simulink model "PSO_MPPT"  (Simulink 10.2)
settings: Solver=FixedStepAuto  StartTime=0.0  StopTime=0.3  FixedStep=1e-6  RelTol=1e-3
undefined symbols (not defined in the file): L
libraries: powerlib x16, re_lib x4, powerlib_meascontrol x1
settings Model: Creator=11383  LastModifiedBy=YiboWang  SimulationMode=accelerator
settings DataIOCC: SaveFormat=Dataset  SignalLoggingSaveFormat=Dataset
settings OptimizationCC: LifeSpan=auto
settings DebuggingCC: UnderspecifiedInitializationDetection=Simplified  MergeDetectMultiDrivingBlocksExec=error  FcnCallInpInsideContextMsg=error  SFUnexpectedBacktrackingDiag=error  SFNoUnconditionalDefaultTransitionDiag=error  SFExecutionAtInitializationDiag=warning
settings HardwareCC: ProdBitPerPointer=64  ProdBitPerSizeT=64  ProdBitPerPtrDiffT=64  ProdLargestAtomicFloat=Float  ProdIntDivRoundTo=Zero  ProdEndianess=LittleEndian  ProdWordSize=64  ProdHWDeviceType=Intel->x86-64 (Windows64)
settings ModelReferenceCC: PropagateSignalLabelsOutOfModel=on
settings GRTTargetCC: TargetLangStandard=C99 (ISO)  CombineOutputUpdateFcns=on  GRTInterface=off
settings ConfigComp: CovMetricSettings=dwe  CovSaveCumulativeToWorkspaceVar=off  CovSaveSingleToWorkspaceVar=off  CovExternalEMLEnable=on
settings SimscapeCC: SimscapeNormalizeSystem=off

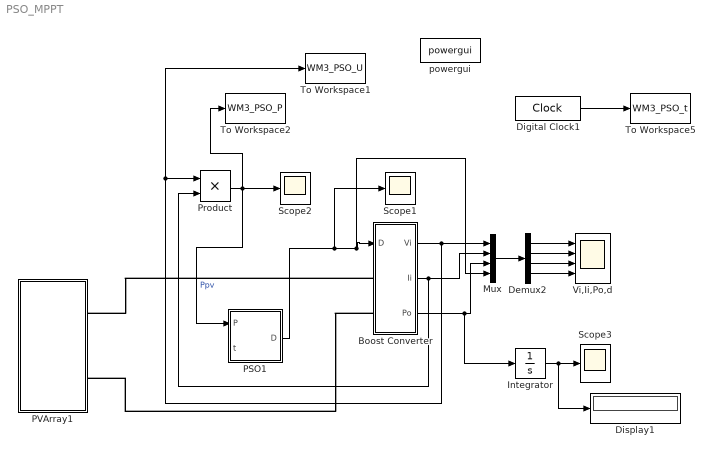
== system PSO_MPPT ==
  Boost Converter : Subsystem
  Demux2 : Demux
  Digital Clock1 : DigitalClock  SampleTime=-1
  Display1 : Display
  Integrator : Integrator
  Mux : Mux
  PSO1 : MATLAB Function  TreatAsAtomicUnit=on  SystemSampleTime=0.005
  PVArray1 : Subsystem
  Product : Product
  Scope1 : Scope
  Scope2 : Scope
  Scope3 : Scope
  To Workspace1 : ToWorkspace  VariableName=WM3_PSO_U  SampleTime=-1
  To Workspace2 : ToWorkspace  VariableName=WM3_PSO_P  SampleTime=-1
  To Workspace5 : ToWorkspace  VariableName=WM3_PSO_t  SampleTime=-1
  Vi,Ii,Po,d : Scope  NumInputPorts=4
  powergui : powerlib/powergui  SimulationMode=Discrete  SampleTime=1e-6  frequency=60  Iterations=50  frequencyindice=0  Pbase=100e6  ErrMax=1e-4  UnitsV=kV  UnitsW=MW  buscounter=0  FunctionMessages=off  echomessages=off  EnableUseOfTLC=off  CurrentSourceSwitches=off  DisableSnubberDevices=off  DisableRonSwitches=off  DisableVfSwitches=off  DisplayEquations=off  AutomaticDiscreteSolvers=off  SolverType=Tustin  Interpol=off  ExternalGateDelay=off  methode=off  Ts=0  x0status=blocks  SPID=off  SwTol=0  HookPort=off  NonlinearTolerance=0  nMaxIteration=15  ContinueOnMaxIteration=off  RestoreLinks=warning  ResistiveCurrentMeasurement=off  Frange=[0:2:500]  Ylog=off  Xlog=on  ShowGrid=off  save=off  variable=ZData  structure=0  ZoomFFT=on  StartTime=0.0  cycles=1  DisplayStyle=1  fundamental=60  FreqAxis=off  MaxFrequency=1000  frequencyindicesteady=1  RmsSteady=1  display=off
  wires:
  Digital Clock1/1 -> To Workspace5/1
  Demux2/1 -> Vi,Ii,Po,d/1
  Demux2/2 -> Vi,Ii,Po,d/2
  Demux2/3 -> Vi,Ii,Po,d/3
  Demux2/4 -> Vi,Ii,Po,d/4
  Boost Converter/1(Vi) -> Mux/1, To Workspace1/1, Product/1
  Boost Converter/2(Ii) -> Mux/2, Product/2
  Boost Converter/3(Po) -> Integrator/1, Mux/3
  PSO1/1(D) -> Scope1/1, Mux/4, Boost Converter/1(D)
  Product/1 -> PSO1/1(P), To Workspace2/1, Scope2/1  "Ppv"
  Mux/1 -> Demux2/1
  Integrator/1 -> Display1/1, Scope3/1
  connections:
  Boost Converter/LConn2 -- PVArray1/RConn2
  Boost Converter/LConn1 -- PVArray1/RConn1

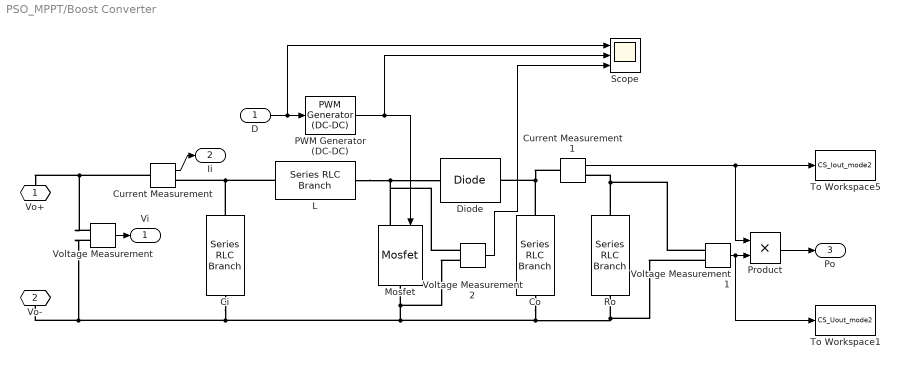
== system PSO_MPPT/Boost Converter ==
  D : Inport
  Ci : powerlib/Elements/Series RLC Branch  LConnTagsString=__new0  RConnTagsString=__new0  BranchType=C  Resistance=1  Inductance=L  SetiL0=off  InitialCurrent=0  Capacitance=10e-5  Setx0=off  InitialVoltage=0  Measurements=None
  Co : powerlib/Elements/Series RLC Branch  LConnTagsString=__new0  RConnTagsString=__new0  BranchType=C  Resistance=1  Inductance=L  SetiL0=off  InitialCurrent=0  Capacitance=9e-05  Setx0=off  InitialVoltage=0  Measurements=None
  Current Measurement : powerlib/Measurements/Current Measurement  PhasorSimulation=off  OutputType=Complex  PSBequivalent=0
  Current Measurement1 : powerlib/Measurements/Current Measurement  PhasorSimulation=off  OutputType=Complex  PSBequivalent=0
  Diode : powerlib/Power Electronics/Diode  Ron=0.001  Lon=0  Vf=0.8  IC=0  UseSnubber=off  Rs=inf  Cs=250e-9  Measurements=off
  L : powerlib/Elements/Series RLC Branch  LConnTagsString=__new0  RConnTagsString=__new0  BranchType=L  Resistance=1  Inductance=2e-3  SetiL0=off  InitialCurrent=0  Capacitance=1e-6  Setx0=off  InitialVoltage=0  Measurements=None
  Mosfet : powerlib/Power Electronics/Mosfet  Ron=0.1  Lon=0  Rd=0.01  Vfd=0  IC=0  Rs=1e5  Cs=inf  Measurements=off
  PWM Generator (DC-DC) : powerlib_meascontrol/Pulse & Signal Generators/PWM Generator (DC-DC)  Fsw=10000  Ts=0
  Product : Product
  Ro : powerlib/Elements/Series RLC Branch  LConnTagsString=__new0  RConnTagsString=__new0  BranchType=R  Resistance=33  Inductance=L  SetiL0=off  InitialCurrent=0  Capacitance=1e-6  Setx0=off  InitialVoltage=0  Measurements=None
  Scope : Scope  NumInputPorts=3
  To Workspace1 : ToWorkspace  VariableName=CS_Uout_mode2  SampleTime=-1
  To Workspace5 : ToWorkspace  VariableName=CS_Iout_mode2  SampleTime=-1
  Voltage Measurement : powerlib/Measurements/Voltage Measurement  PhasorSimulation=off  OutputType=Complex  PSBequivalent=0
  Voltage Measurement1 : powerlib/Measurements/Voltage Measurement  PhasorSimulation=off  OutputType=Complex  PSBequivalent=0
  Voltage Measurement2 : powerlib/Measurements/Voltage Measurement  PhasorSimulation=off  OutputType=Complex  PSBequivalent=0
  Vo+ : PMIOPort  Side=Left
  Vo- : PMIOPort  Port=2  Side=Left
  Vi : Outport  VectorParamsAs1DForOutWhenUnconnected=off
  Ii : Outport  Port=2  VectorParamsAs1DForOutWhenUnconnected=off
  Po : Outport  Port=3  VectorParamsAs1DForOutWhenUnconnected=off
  wires:
  Current Measurement1/1 -> To Workspace5/1, Product/1
  Product/1 -> Po/1
  Voltage Measurement1/1 -> To Workspace1/1, Product/2
  Current Measurement/1 -> Ii/1
  PWM Generator (DC-DC)/1 -> Scope/2, Mosfet/1
  D/1 -> Scope/1, PWM Generator (DC-DC)/1
  Voltage Measurement/1 -> Vi/1
  Voltage Measurement2/1 -> Scope/3
  connections:
  Current Measurement1/LConn1 -- Co/LConn1 -- Diode/RConn1
  L/RConn1 -- Voltage Measurement2/LConn1 -- Mosfet/LConn1 -- Diode/LConn1
  L/LConn1 -- Current Measurement/RConn1 -- Ci/LConn1
  Co/RConn1 -- Voltage Measurement1/LConn2 -- Ro/RConn1 -- Ci/RConn1 -- Vo-/RConn1 -- Voltage Measurement/LConn2 -- Voltage Measurement2/LConn2 -- Mosfet/RConn1
  Ro/LConn1 -- Voltage Measurement1/LConn1 -- Current Measurement1/RConn1
  Current Measurement/LConn1 -- Vo+/RConn1 -- Voltage Measurement/LConn1

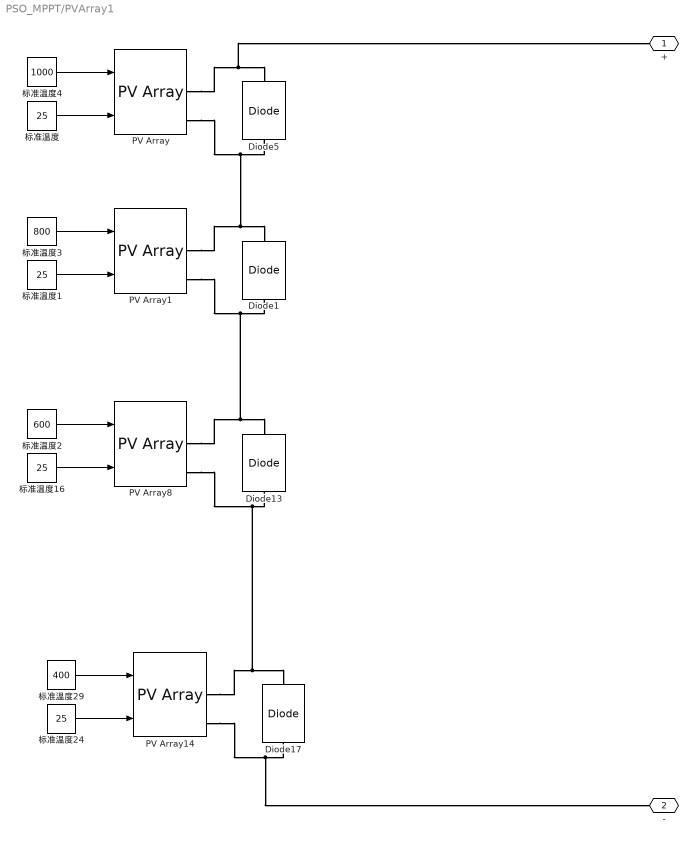
== system PSO_MPPT/PVArray1 ==
  Diode{1,5,13,17} (4 alike) : powerlib/Power Electronics/Diode  Ron=0.001  Lon=0  Vf=0.8  IC=0  UseSnubber=off  Rs=inf  Cs=250e-9  Measurements=off
  PV Array{,1,8,14} (4 alike) : re_lib/Solar/PV Array  Npar=1  Nser=1  PlotType=array @ 1000 W/m2 & specified temperatures  S_vec="[ 1000  500  100 ]"  Temp_C_vec="[ 45 25  ]"  ModuleName=User-defined  PlotWhenSelected=off  Pm=120.75  Ncell=16  Voc=22  Isc=7.5  Vm=17.5  Im=6.9  beta_Voc_pc=-0.36099  alpha_Isc_pc=0.102  beta_Voc=-0.079418  alpha_Isc=0.00765  IL=7.6829  I0=2.1898e-10  nI=2.2089  Rsh=50.0358  Rs=0.26399  RobustModel=off  RobustCellTemperature=313.3991  BAL=off  Tc=1e-6  Tfilter=5e-5
  标准温度{,1,16,24} (4 alike) : Constant  Value=25  SampleTime=0.001
  标准温度2 : Constant  Value=600  SampleTime=0.001
  标准温度29 : Constant  Value=400  SampleTime=0.001
  标准温度3 : Constant  Value=800  SampleTime=0.001
  标准温度4 : Constant  Value=1000  SampleTime=0.001
  + : PMIOPort  Side=Right
  - : PMIOPort  Port=2  Side=Right
  wires:
  标准温度16/1 -> PV Array8/2
  标准温度24/1 -> PV Array14/2
  标准温度29/1 -> PV Array14/1
  标准温度1/1 -> PV Array1/2
  标准温度/1 -> PV Array/2
  标准温度2/1 -> PV Array8/1
  标准温度3/1 -> PV Array1/1
  标准温度4/1 -> PV Array/1
  connections:
  Diode17/RConn1 -- PV Array14/RConn1 -- Diode13/LConn1 -- PV Array8/RConn2
  Diode5/RConn1 -- +/RConn1 -- PV Array/RConn1
  Diode5/LConn1 -- PV Array/RConn2 -- Diode1/RConn1 -- PV Array1/RConn1
  Diode17/LConn1 -- -/RConn1 -- PV Array14/RConn2
  Diode13/RConn1 -- PV Array8/RConn1 -- Diode1/LConn1 -- PV Array1/RConn2

== matlab function PSO1 ==
  data: D output double; P input double; t input double
function D=PSO(P,t)
%% 参数定义
w=0.5;                              %惯性权重
c1=0.5;                             %个体学习因子/加速度因子
c2=0.9;                             %群体学习因子/加速度因子
N=4;                                %粒子个数
pmin=0.1;                           %输出最小值
pmax=0.9;                             %输出最大值
r1=rand;
r2=rand;
%% Starting Up
persistent p;
if isempty(p) 
    %Create empty particle 定义空粒子属性
    %p.x=[0.1 0.25 0.4 0.55 0.7];
    %p.x=[0.1 0.3 0.5 0.7];
    p.x=[0.1,0.3,0.6,0.9];
    %p.x = linspace(0.4,0.6,N);
    %p.x = linspace(pmin,pmax,N);    %线性平均划分输出的最小最大差值成为N个数
    p.v = zeros(1,N);               %粒子速度初始化
    p.y = zeros(1,N);               %粒子位置对应值初始化
	p.bx = zeros(1,N);              %粒子最优位置初始化
    p.by = zeros(1,N);              %粒子最优值初始化
    p.bg=pmin;                      %全局最优值初始化
    p.k=1;                          %控制循环次数
    D=p.x(p.k);                     %输出值初始化
else
%% Input
p.y(p.k)=P;                         %存储输入的功率值到p.y中的第p.k个

%% Best Particle 寻找最优粒子
if p.y(p.k)>p.by(p.k)               %如果某一点的P值大于最优值的话
    p.bx(p.k)=p.x(p.k);             %把更高的P值对应的电压值赋给最优值
    p.by(p.k)=p.y(p.k);             %把更高的P值赋给最优值
end


%% PSO算法
p.v(p.k)=w*p.v(p.k)+c1*r1*(p.bx(p.k)-p.x(p.k))+c2*r2*(p.bg-p.x(p.k));%速度更新,p.k控制粒子顺序
p.x(p.k)=p.x(p.k)+p.v(p.k);         %位置更新
%% 输出限幅
if p.x(p.k)<=pmin
   p.x(p.k)=pmin;
end
if p.x(p.k)>=pmax
    p.x(p.k)=pmax;
end
%% Update Particle Turn,k 更新循环次数
p.k=p.k+1;
if p.k>N                            %当每个粒子都进行循环后，p.k超过N，则比较目前得到的功率P值
    [a,b]=max(p.by);                %a为最大值，b为最大值的索引，p.by为P最大值
    p.bg=p.bx(b);                   %p.bx为之前过程中的最高P值，b为所有最高值中的最高值，p.bg为目前最大P
    p.k=1;                          %p.k回1，重新循环
end
%% Output 输出到PWM
D=p.x(p.k);                         %输出为4个粒子对应的D值
end
